simulink model "UAV2018NLObs"  (R2021a)
settings: Solver=FixedStepAuto  StartTime=0.0  StopTime=5  FixedStep=0.1  RelTol=1e-6  EnableMultiTasking=on
values from neighbouring files (symbols this model uses):
  control_lb = [0.01;-0.5]    [prueba.m]
  control_ub = [1.1;0.5]    [prueba.m]
  fc = [21;0;0;0]    [prueba.m]
  Kd = K(5:6)    [prueba.m]
  Ki = K(3:4)    [prueba.m]
  Kp = K(1:2)    [prueba.m]
  refer = 20    [prueba.m]
  x0 = [-1;0;0.05;0]    [Calculos20.m]
undefined symbols (not defined in the file or in its folder): Xtrim
settings Model: PacingRate=0.790000  Creator=Ignacio  LastModifiedBy=Pablo
settings SolverCC: AlgebraicLoopSolver=TrustRegion
settings DataIOCC: LimitDataPoints=on  SaveFormat=Array  ReturnWorkspaceOutputs=off
settings OptimizationCC: ExpressionDepthLimit=2147483647  LifeSpan=inf
settings DebuggingCC: UnderspecifiedInitializationDetection=Classic  MergeDetectMultiDrivingBlocksExec=none  FcnCallInpInsideContextMsg=warning  StateNameClashWarn=warning  SFUnexpectedBacktrackingDiag=warning  SFNoUnconditionalDefaultTransitionDiag=warning  SFExecutionAtInitializationDiag=none  SFMachineParentedDataDiag=warning  ArithmeticOperatorsInVariantConditions=warning
settings HardwareCC: ProdBitPerPointer=32  ProdBitPerSizeT=32  ProdBitPerPtrDiffT=32  ProdLargestAtomicFloat=None  ProdIntDivRoundTo=Undefined  ProdEndianess=Unspecified  ProdWordSize=32  ProdHWDeviceType=32-bit Generic
settings ModelReferenceCC: PropagateSignalLabelsOutOfModel=off
settings SFSimCC: SimUseLocalCustomCode=off  CustomCodeUndefinedFunction=UseInterfaceOnly
settings RTWCC: RTWUseLocalCustomCode=off
settings CodeAppCC: StateflowObjectComments=on
settings GRTTargetCC: TargetLangStandard=C89/C90 (ANSI)
settings ConfigComp: CovMetricSettings=dw  CovSaveCumulativeToWorkspaceVar=on  CovSaveSingleToWorkspaceVar=on  CovExternalEMLEnable=off

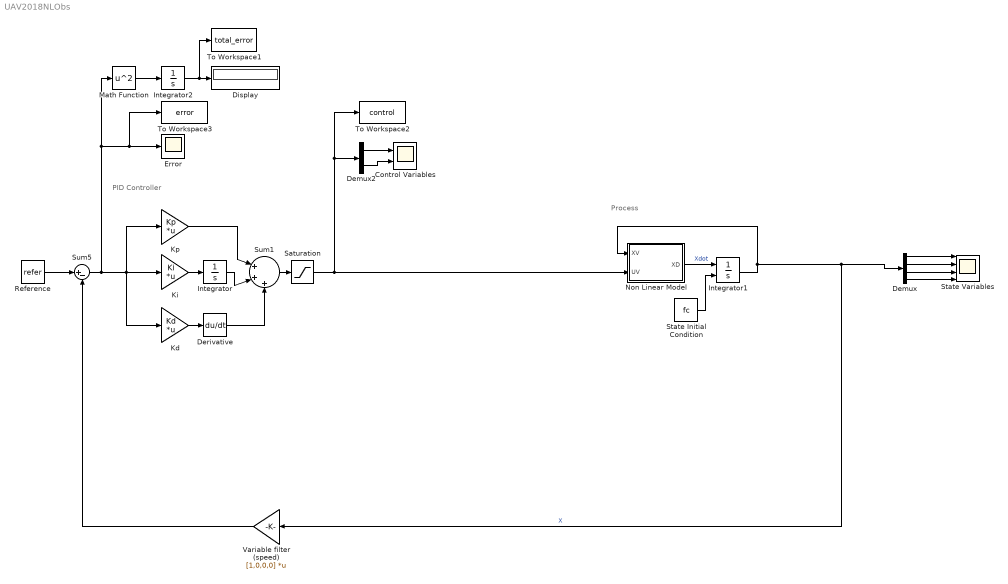
== system UAV2018NLObs ==
  note: Process
  note: PID Controller
  " Non Linear Model" : MATLAB Function  TreatAsAtomicUnit=on
  Control Variables : Scope  NumInputPorts=2
  Demux : Demux
  Demux2 : Demux  Outputs=2
  Derivative : Derivative
  Display : Display
  Error : Scope
  Integrator : Integrator
  Integrator1 : Integrator  InitialConditionSource=external  InitialCondition=Xtrim+x0
  Integrator2 : Integrator
  Kd : Gain  Gain=Kd  Multiplication=Matrix(K*u)
  Ki : Gain  Gain=Ki  Multiplication=Matrix(K*u)
  Kp : Gain  Gain=Kp  Multiplication=Matrix(K*u)
  Math Function : Math  Operator=square  SaturateOnIntegerOverflow=on
  Reference : Constant  Value=refer
  Saturation : Saturate  UpperLimit=control_ub  LowerLimit=control_lb  ZeroCross=off
  State Initial Condition : Constant  Value=fc
  State Variables : Scope  NumInputPorts=4
  Sum1 : Sum  Inputs=|+++
  Sum5 : Sum  Inputs=|+-
  To Workspace1 : ToWorkspace  VariableName=total_error  SampleTime=-1
      settings: MaxDataPoints=1
  To Workspace2 : ToWorkspace  VariableName=control  SampleTime=-1
  To Workspace3 : ToWorkspace  VariableName=error  SampleTime=-1
  Variable filter (speed) : Gain  Gain=[1,0,0,0]  Multiplication=Matrix(K*u)
  wires:
  Demux/4 -> State Variables/4
  Demux/3 -> State Variables/3
  Demux/2 -> State Variables/2
  Demux/1 -> State Variables/1
  Demux2/2 -> Control Variables/2
  Demux2/1 -> Control Variables/1
  Integrator1/1 -> Variable filter (speed)/1, Demux/1, " Non Linear Model"/1(XV)  "X"
  " Non Linear Model"/1(XD) -> Integrator1/1  "Xdot"
  State Initial Condition/1 -> Integrator1/2
  Variable filter (speed)/1 -> Sum5/2
  Reference/1 -> Sum5/1
  Ki/1 -> Integrator/1
  Kd/1 -> Derivative/1
  Derivative/1 -> Sum1/3
  Integrator/1 -> Sum1/2
  Kp/1 -> Sum1/1
  Sum5/1 -> Kd/1, Kp/1, Ki/1, Math Function/1, To Workspace3/1, Error/1
  Sum1/1 -> Saturation/1
  Saturation/1 -> To Workspace2/1, Demux2/1, " Non Linear Model"/2(UV)
  Integrator2/1 -> To Workspace1/1, Display/1
  Math Function/1 -> Integrator2/1

== matlab function UAV2018NLObs/ Non Linear Model ==
  data: XV input; XD output; UV input
function XD = UAVNL(XV,UV)

% Modelo dinámico del UAV. Dinámica longitudinal.
% Esta función calcula el vector derivadas de las variables de estado a 
% partir del vector del estado y el vector de control

% versión 2014:con Vt y Alpha y motor instantaneo
% versión 2016: con XCG como entrada
% versión 2018: Eliminados X y Z. XCG Fijo


XD=zeros(4,1); % Inicializamos el vector de las derivadas con ceros

% DATOS DE LA AERONAVE

S = 0.4121;               % superficie alar (m^2)
C=0.2192;                  % cuerda media aerodinámica (m)
MASA=2.5;                  % Masa (Kg)
XCGR=0.33;                % posición de referencia del CG
IP=0.156794;                   % Momento de inercia (Kg*m^2)
d=1.225;                      % densidad (Kg/m^3)
G=9.8;                    % gravedad m/s^2
XCG=.33;                  % CG coincide con el de referencia

% derivadas de estabilidad y control adimensionales

CLalpha0=0.405;    
CLalpha=5.379292;
CLq=11.133615;
CD0=0.0277;
CDalpha=0.14897;
CDalpha2=0.9848;
Cm0=0.0418;     
Cmalpha=-1.812981; 
Cmalphadot=-7.0;
Cmde=-1.552;
Cmq=-18.422237;

% variables de estado

VT=XV(1);	% Velocidad 
ALPHA=XV(2);	% Angulo de ataque
THETA=XV(3);% Angulo de asiento
Q=XV(4);	% Velocidad angular de cabeceo


% variables de control

Dt=UV(1);	% Acelerador
De=UV(2);	% Deflexión del timón de profundidad

% Algunos calculos previos

U=VT*cos(ALPHA);	% Componentes de la velocidad en ejes cuerpo
W=VT*sin(ALPHA);	

PDS=0.5*d*(VT^2)*S;	% Presión dinámica*Superficie alar

% Parametros Grupo Motopropulsor

Dh=0.254;   % Diametro de la helice (m)

REVmax=222; % Revoluciones maximas del motor (rev/s)

CT0=0.13805; % Coeficientes de traccion
CTj=-0.2049;
REV=REVmax*Dt; % Motor instantaneo
J=VT/(REV*Dh);  %Coef de velocidad
C_T=CT0+CTj*J;          %Coef de traccion
T=C_T*d*REV^2*Dh^4;     %Traccion

% coeficientes adimensionales de fuerzas y momentos (ejes viento)

CLT=CLalpha0+CLalpha*ALPHA+CLq*Q*C*0.5/VT;         
CDT=CD0+CDalpha*ALPHA+CDalpha2*ALPHA^2;  
CZ=-CDT*sin(ALPHA)-CLT*cos(ALPHA); % Cz en ejes cuerpo para añadir despues el efecto del centro de gravedad
CmT=Cm0+(Cmalpha*ALPHA)+(Cmde*De)+(CZ*(XCG-XCGR))+(C*0.5*Cmq*Q/VT); % Falta la componente alphadot,la añadiremos despues

% Fuerzas aerodinámicas

L=CLT*PDS;
D=CDT*PDS;

% Sistema de ecuaciones diferenciales de la dinámica del vuelo

%XDOT=cos(THETA)*U+sin(THETA)*W;
%ZDOT=sin(THETA)*U-cos(THETA)*W; %Esto realmente no es z, le he cambiado el signo y es altitud
UDOT=-Q*W+(T-MASA*G*sin(THETA)-D*cos(ALPHA)+L*sin(ALPHA))/MASA;
WDOT=Q*U+(MASA*G*cos(THETA)-D*sin(ALPHA)-L*cos(ALPHA))/MASA;
ALPHADOT=((U*WDOT-W*UDOT)/VT^2);
CmT=CmT+Cmalphadot*C/(2*VT)*ALPHADOT; % Completamos Cm
QDOT=CmT*PDS*C/IP;

VTDOT=(U*UDOT+W*WDOT)/VT;

% Construimos el vector con las derivadas de las variables de estado


XD(1)=VTDOT;
XD(2)=ALPHADOT;
XD(3)=Q;
XD(4)=QDOT;
